simulink model "arm_sim"  (R2019b)
settings: Solver=ode45  StartTime=0.0  StopTime=10000  RelTol=1e-3  EnableMultiTasking=on
InitFcn:
  | addpath ./..
  | armParam
undefined symbols (not defined in the file): drawArm, P
libraries: simulink x1
settings Model: Creator=beard  LastModifiedBy=JoHn
settings DataIOCC: LimitDataPoints=on  SaveFormat=Array  SignalLoggingSaveFormat=ModelDataLogs  ReturnWorkspaceOutputs=off
settings OptimizationCC: ExpressionDepthLimit=2147483647  InitFltsAndDblsToZero=on  LifeSpan=inf
settings DebuggingCC: UnderspecifiedInitializationDetection=Classic  MergeDetectMultiDrivingBlocksExec=none  SolverPrmCheckMsg=warning  FcnCallInpInsideContextMsg=warning  StateNameClashWarn=warning  SFUnexpectedBacktrackingDiag=warning  SFNoUnconditionalDefaultTransitionDiag=warning  SFExecutionAtInitializationDiag=none  ArithmeticOperatorsInVariantConditions=warning
settings HardwareCC: ProdBitPerPointer=32  ProdBitPerSizeT=32  ProdBitPerPtrDiffT=32  ProdLargestAtomicFloat=None  ProdIntDivRoundTo=Undefined  ProdEndianess=Unspecified  ProdWordSize=32  ProdHWDeviceType=32-bit Generic
settings ModelReferenceCC: PropagateSignalLabelsOutOfModel=off
settings SFSimCC: SimUseLocalCustomCode=off  CustomCodeUndefinedFunction=UseInterfaceOnly
settings RTWCC: RTWUseLocalCustomCode=off
settings CodeAppCC: StateflowObjectComments=on
settings GRTTargetCC: TargetLangStandard=C89/C90 (ANSI)  GeneratePreprocessorConditionals=Disable all  CombineOutputUpdateFcns=off  GRTInterface=on
settings ConfigComp: CovMetricSettings=dw  CovHtmlReporting=on  CovSaveCumulativeToWorkspaceVar=on  CovSaveSingleToWorkspaceVar=on  CovExternalEMLEnable=off

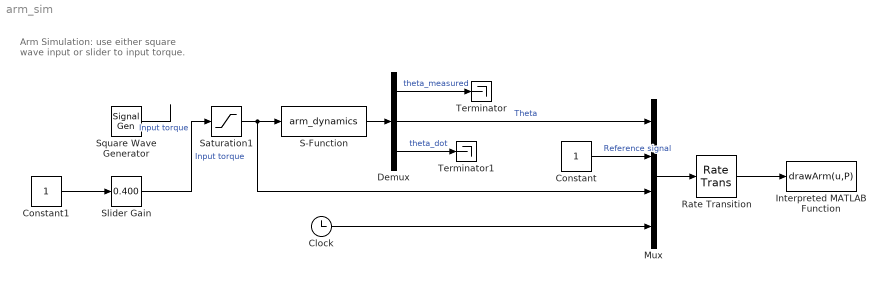
== system arm_sim ==
  note: Arm Simulation: use either
      | square wave input or slider
      | to input torque.
  Clock : Clock
  Constant : Constant
  Constant1 : Constant
  Demux : Demux  Outputs=[1,1,1]
  Interpreted MATLAB Function : MATLABFcn  MATLABFcn=drawArm(u,P)  OutputDimensions=0
  Mux : Mux
  Rate Transition : RateTransition  OutPortSampleTime=P.t_plot
  S-Function : S-Function  FunctionName=arm_dynamics  Parameters=P  SFunctionDeploymentMode=off  EnableBusSupport=off
  Saturation1 : Saturate  UpperLimit=P.tau_max  LowerLimit=-P.tau_max
  Slider Gain : simulink/Math Operations/Slider Gain  gain=0.400  low=-1  high=1
  Square Wave Generator : SignalGenerator  WaveForm=square  Amplitude=.2  Frequency=.5  Units=rad/sec
  Terminator : Terminator
  Terminator1 : Terminator
  wires:
  Square Wave Generator/1 -> ?  "Input torque"
  Saturation1/1 -> Mux/3, S-Function/1
  Constant/1 -> Mux/2  "Reference signal"
  Clock/1 -> Mux/4
  Mux/1 -> Rate Transition/1
  Rate Transition/1 -> Interpreted MATLAB Function/1
  Constant1/1 -> Slider Gain/1
  Slider Gain/1 -> Saturation1/1  "Input torque"
  S-Function/1 -> Demux/1
  Demux/1 -> Terminator/1  "theta_measured"
  Demux/2 -> Mux/1  "Theta"
  Demux/3 -> Terminator1/1  "theta_dot"
